simulink model "Wander_Panacea43_1"  (R2019b)
settings: Solver=VariableStepAuto  StartTime=0.0  StopTime=0.5  RelTol=1e-3
values from neighbouring files (symbols this model uses):
  Q = diag([1e-5 1e-5 3])    [panacea_odet.m]    (also in panacea_odet_b.m = diag([1e-2 1e-2 6]); test_kf_simple.m = 0.5)
  R = 0.5*eye(3)    [panacea_odet.m]    (also in panacea_odet_b.m = 0.005*eye(3); test_kf_simple.m = 0.2)
  z = zeros(length(ofdx)*2+3*tracking_delay_length,1,length(out.ofd.time))    [panacea_1.m]    (also in panacea_2.m = zeros(length(ofdx)*2+3*tracking_delay_length+6,1); panacea_3.m = zeros(length(ofdx)*2+3*tracking_delay_length+6,1); panacea_4.m = zeros(length(ofdx)*2+3*tracking_delay_length+6,1); panacea_5.m = zeros(length(ofdx)*2+3*tracking_delay_length+6,1))
undefined symbols (not defined in the file or in its folder): Aa, Add, Ba, Bdd, Cdd, DiscIntNeverNeededParam, f, imuTs, lms, numOfLm, phi, psi, the, x, y
libraries: simulink x9, sharedtransform x2, dspswit3 x1
settings Model: Creator=thinhhoang  LastModifiedBy=thinhhoang
settings OptimizationCC: DefaultParameterBehavior=Inlined  EnhancedBackFolding=on  PassReuseOutputArgsAs=Individual arguments  ZeroExternalMemoryAtStartup=off  ZeroInternalMemoryAtStartup=off  OptimizeBlockOrder=speed  DifferentSizesBufferReuse=on  OptimizationCustomize=off  EfficientTunableParamExpr=on
settings DebuggingCC: ParameterTunabilityLossMsg=error
settings SFSimCC: MATLABDynamicMemAlloc=off
settings RTWCC: SystemTargetFile=ert.tlc  TemplateMakefile=ert_default_tmf  GenerateReport=on  IncludeHyperlinkInReport=on  LaunchReport=on  GenerateTraceInfo=on  GenerateTraceReport=on  GenerateTraceReportSl=on  GenerateTraceReportSf=on  GenerateTraceReportEml=on
settings CodeAppCC: ForceParamTrailComments=on  IgnoreCustomStorageClasses=off  OperatorAnnotations=on  SimulinkDataObjDesc=on  SFDataObjDesc=on  InsertBlockDesc=on
settings ERTTargetCC: TargetLangStandard=C99 (ISO)  GenerateSampleERTMain=on  InlinedParameterPlacement=NonHierarchical  ERTCustomFileTemplate=example_file_process.tlc

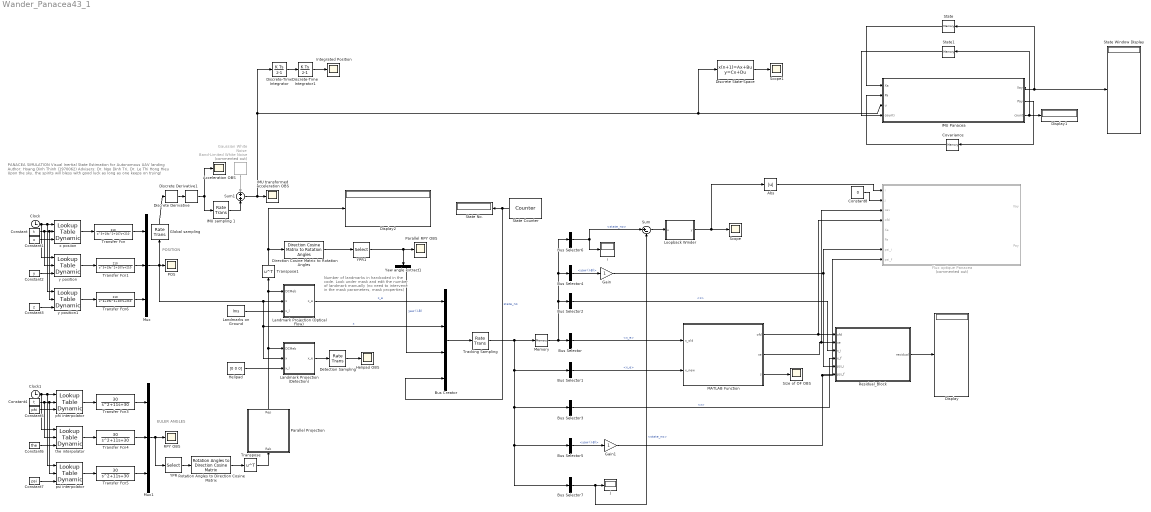
== system Wander_Panacea43_1 ==
  note: PANACEA SIMULATION
      | Visual Inertial State Estimation for Autonomous UAV landing
      | Author: Hoang Dinh Thinh (1970062)
      | Advisers: Dr. Ngo Dinh Tri, Dr. Le Thi Hong Hieu
      | Upon the sky, the spirits will bless with good luck as long as
      | one keeps on trying!
  note: Number of landmarks in hardcoded in the code. Look under mask and edit the number of landmark manually (no need to intervene in the mask parameters, mask properties)
  note: POSITION
  note: EULER ANGLES
  Abs : Abs
  Acceleration OBS : Scope
  Bus Creator : BusCreator  Inputs=4
  Bus Selector : BusSelector  OutputSignals=x_e
  Bus Selector1 : BusSelector  OutputSignals=x_e
  Bus Selector2 : BusSelector  OutputSignals=x
  Bus Selector3 : BusSelector  OutputSignals=x
  Bus Selector4 : BusSelector  OutputSignals=yaw (I-B)
  Bus Selector5 : BusSelector  OutputSignals=yaw (I-B)
  Bus Selector6 : BusSelector  OutputSignals=state_no
  Bus Selector7 : BusSelector  OutputSignals=state_no
  Clock : Clock
  Clock1 : Clock
  Constant : Constant  Value=t
  Constant1 : Constant  Value=x
  Constant2 : Constant  Value=y
  Constant3 : Constant  Value=z
  Constant4 : Constant  Value=t
  Constant5 : Constant  Value=phi
  Constant6 : Constant  Value=the
  Constant7 : Constant  Value=psi
  Constant8 : Constant  Value=0
  Covariance : Memory  InitialCondition=zeros(6,6)
  "Detection Sampling " : RateTransition  OutPortSampleTime=detectionTs
  Direction Cosine Matrix to Rotation Angles : sharedtransform/Direction Cosine Matrix to Rotation Angles  rotationOrder=ZYX  aMode=aMode  action=None  tolerance=eps(2)
      settings: SourceProductName=Aerospace Blockset  SourceProductBaseCode=AE
  Discrete Derivative : simulink/Quick Insert/Discrete/Discrete Derivative  gainval=1.0  ICPrevScaledInput=0.0  OutMin=[]  OutMax=[]  OutDataType=fixdt(1, 16)  OutScaling=2^-10  DoSatur=off
      settings: SourceProductName=Simulink  SourceProductBaseCode=SL
  Discrete Derivative1 : simulink/Quick Insert/Discrete/Discrete Derivative  gainval=1.0  ICPrevScaledInput=0.0  OutMin=[]  OutMax=[]  OutDataType=fixdt(1, 16)  OutScaling=2^-10  DoSatur=off
      settings: SourceProductName=Simulink  SourceProductBaseCode=SL
  Discrete State-Space : DiscreteStateSpace  A=Add  B=Bdd  C=Cdd  D=zeros(3)  SampleTime=-1
  Discrete-Time Integrator : DiscreteIntegrator  SampleTime=-1  ICPrevOutput=DiscIntNeverNeededParam  ICPrevScaledInput=DiscIntNeverNeededParam
  Discrete-Time Integrator1 : DiscreteIntegrator  SampleTime=-1  ICPrevOutput=DiscIntNeverNeededParam  ICPrevScaledInput=DiscIntNeverNeededParam
  Display : Display
  Display1 : Display
  Display2 : Display
  Flux optique Panacea : MATLAB Function  Commented=on  TreatAsAtomicUnit=on  mask{Q=Q, R=R, f=f, Aa=Aa, Ba=Ba}
  Gain : Gain
  Gain1 : Gain
  Gaussian White Noise : simulink/Sources/Band-Limited White Noise  Commented=on  Cov=[1e-3]  Ts=imuTs  seed=[23341]
  Global sampling : RateTransition  OutPortSampleTime=globalTs
  Helipad : Constant  Value=[0 0 0]
  Helipad OBS : Scope
  IMU Panacea : MATLAB Function  TreatAsAtomicUnit=on  SystemSampleTime=imuTs  mask{Q=Q, Aa=Add, Ba=Bdd}
  IMU sampling 1 : RateTransition  OutPortSampleTime=imuTs
  IMU transformed acceleration OBS : Scope
  Integrated Position : Scope
  Landmark Projection (Detection) : MATLAB Function  TreatAsAtomicUnit=on  mask{f=f, numOfLm=1}
      mask prompts: f "Focal length"; numOfLm "Number of landmarks"
  Landmark Projection (Optical Flow) : MATLAB Function  TreatAsAtomicUnit=on  mask{f=f, numOfLm=numOfLm}
      mask prompts: f "Focal length"; numOfLm "Number of landmarks"
  Landmarks on Ground : Constant  Value=lms
  Loopback Winder : MATLAB Function  TreatAsAtomicUnit=on
  MATLAB Function : MATLAB Function  TreatAsAtomicUnit=on
  Memory : Memory  InheritSampleTime=on
  Mux : Mux  Inputs=3
  Mux1 : Mux  Inputs=3
  POS : Scope
  Parallel Projection : MATLAB Function  TreatAsAtomicUnit=on
  Parallel RPY OBS : Scope
  RPY OBS : Scope
  Residual_Block : MATLAB Function  TreatAsAtomicUnit=on  mask{f=f, numOfLm=numOfLm}
      mask prompts: f "Focal length"; numOfLm "Num of LM"
  Rotation Angles to Direction Cosine Matrix : sharedtransform/Rotation Angles to Direction Cosine Matrix  rotationOrder=ZYX  aMode=aMode
      settings: SourceProductBaseCode=AE
  Scope : Scope
  Scope1 : Scope
  Size of OF OBS : Scope
  State : Memory  InitialCondition=zeros(6,1)
  State Counter : dspswit3/Counter  Direction=Up  CountEvent=Free running  CounterSize=User defined  MaxCount=3  InitialCount=0  Output=Count  HitValue=32  ResetInput=on  SamplesPerFrame=1  Ts=imuTs  CntDtype=double  HitDtype=Logical
  State No. : Display
  State Window Display : Display
  State1 : Memory
  Sum : Sum  Inputs=|+-
  Sum1 : Sum  Inputs=+|+
  Tracking Sampling : RateTransition  OutPortSampleTime=trackingTs
  Transfer Fcn : TransferFcn  Numerator=[210]  Denominator=[1 19 107 210]
  Transfer Fcn1 : TransferFcn  Numerator=[210]  Denominator=[1 19 107 210]
  Transfer Fcn3 : TransferFcn  Numerator=[30]  Denominator=[1 11 30]
  Transfer Fcn4 : TransferFcn  Numerator=[30]  Denominator=[1 11 30]
  Transfer Fcn5 : TransferFcn  Numerator=[30]  Denominator=[1 11 30]
  Transfer Fcn6 : TransferFcn  Numerator=[210]  Denominator=[1 19 107 210]
  Transpose : Math  Operator=transpose  SignedPower=off  SaturateOnIntegerOverflow=on
  Transpose1 : Math  Operator=transpose  SignedPower=off  SaturateOnIntegerOverflow=on
  YPR : Selector  InputPortWidth=3  IndexOptions=Index vector (dialog)  Indices=[3 2 1]  OutputSizes=1
  YPR1 : Selector  InputPortWidth=3  IndexOptions=Index vector (dialog)  Indices=[3 2 1]  OutputSizes=1
  Yaw angle extract1 : Demux  Outputs=3
  i : Display
  j : Display
  phi interpolator : simulink/Lookup Tables/Lookup Table Dynamic  LookUpMeth=Interpolation-Use End Values  OutDataType=fixdt('double')  OutScaling=[]  OutputDataTypeScalingMode=Specify via dialog  OutDataTypeStr=double  DoSatur=off
      settings: SourceProductName=Simulink
  psi interpolator : simulink/Lookup Tables/Lookup Table Dynamic  LookUpMeth=Interpolation-Use End Values  OutDataType=fixdt('double')  OutScaling=[]  OutputDataTypeScalingMode=Specify via dialog  OutDataTypeStr=double  DoSatur=off
      settings: SourceProductName=Simulink
  the interpolator : simulink/Lookup Tables/Lookup Table Dynamic  LookUpMeth=Interpolation-Use End Values  OutDataType=fixdt('double')  OutScaling=[]  OutputDataTypeScalingMode=Specify via dialog  OutDataTypeStr=double  DoSatur=off
      settings: SourceProductName=Simulink
  x posiion : simulink/Lookup Tables/Lookup Table Dynamic  LookUpMeth=Interpolation-Use End Values  OutDataType=fixdt('double')  OutScaling=[]  OutputDataTypeScalingMode=Specify via dialog  OutDataTypeStr=double  DoSatur=off
      settings: SourceProductName=Simulink
  y position : simulink/Lookup Tables/Lookup Table Dynamic  LookUpMeth=Interpolation-Use End Values  OutDataType=fixdt('double')  OutScaling=[]  OutputDataTypeScalingMode=Specify via dialog  OutDataTypeStr=double  DoSatur=off
      settings: SourceProductName=Simulink
  y position1 : simulink/Lookup Tables/Lookup Table Dynamic  LookUpMeth=Interpolation-Use End Values  OutDataType=fixdt('double')  OutScaling=[]  OutputDataTypeScalingMode=Specify via dialog  OutDataTypeStr=double  DoSatur=off
      settings: SourceProductName=Simulink
  wires:
  Clock/1 -> y position/1, y position1/1, x posiion/1
  Constant/1 -> y position/2, y position1/2, x posiion/2
  Constant1/1 -> x posiion/3
  Constant2/1 -> y position/3
  Constant3/1 -> y position1/3
  x posiion/1 -> Transfer Fcn/1
  Transfer Fcn/1 -> Mux/1
  Mux/1 -> Global sampling/1, Landmark Projection (Detection)/2(x), Bus Creator/2, Landmark Projection (Optical Flow)/2(x), POS/1  "x"
  Clock1/1 -> the interpolator/1, psi interpolator/1, phi interpolator/1
  Constant4/1 -> the interpolator/2, psi interpolator/2, phi interpolator/2
  Constant5/1 -> phi interpolator/3
  Constant6/1 -> the interpolator/3
  Constant7/1 -> psi interpolator/3
  phi interpolator/1 -> Transfer Fcn3/1
  the interpolator/1 -> Transfer Fcn4/1
  psi interpolator/1 -> Transfer Fcn5/1
  Transfer Fcn3/1 -> Mux1/1
  Transfer Fcn4/1 -> Mux1/2
  Transfer Fcn5/1 -> Mux1/3
  Mux1/1 -> YPR/1, RPY OBS/1
  YPR/1 -> Rotation Angles to Direction Cosine Matrix/1
  Rotation Angles to Direction Cosine Matrix/1 -> Transpose/1
  Landmarks on Ground/1 -> Landmark Projection (Optical Flow)/3(x_l)
  Transpose/1 -> Parallel Projection/1(Reb)
  Parallel Projection/1(Rep) -> Landmark Projection (Detection)/1(DCMeb), Landmark Projection (Optical Flow)/1(DCMeb), Transpose1/1
  Transpose1/1 -> Display2/1, Direction Cosine Matrix to Rotation Angles/1
  Direction Cosine Matrix to Rotation Angles/1 -> YPR1/1
  YPR1/1 -> Yaw angle extract1/1, Parallel RPY OBS/1
  Discrete Derivative/1 -> Discrete Derivative1/1
  Discrete Derivative1/1 -> IMU sampling 1/1, Acceleration OBS/1
  Transfer Fcn1/1 -> Mux/2
  y position/1 -> Transfer Fcn1/1
  y position1/1 -> Transfer Fcn6/1
  Transfer Fcn6/1 -> Mux/3
  Gaussian White Noise/1 -> Sum1/1
  MATLAB Function/3(s) -> Size of OF OBS/1
  Helipad/1 -> Landmark Projection (Detection)/3(x_l)
  Landmark Projection (Detection)/1(x_e) -> "Detection Sampling "/1
  "Detection Sampling "/1 -> Helipad OBS/1
  IMU sampling 1/1 -> Sum1/2
  Global sampling/1 -> Discrete Derivative/1
  Landmark Projection (Optical Flow)/1(x_e) -> Bus Creator/1  "x_e"
  Bus Creator/1 -> Tracking Sampling/1
  Tracking Sampling/1 -> Bus Selector7/1, Bus Selector5/1, Bus Selector3/1, Bus Selector1/1, Memory/1
  Memory/1 -> Bus Selector6/1, Bus Selector4/1, Bus Selector2/1, Bus Selector/1
  Bus Selector/1 -> MATLAB Function/1(x_old)  "<x_e>"
  Bus Selector1/1 -> MATLAB Function/2(x_new)  "<x_e>"
  MATLAB Function/1(ofd) -> Flux optique Panacea/4(ofd), Residual_Block/1(ofd)
  MATLAB Function/2(xe) -> Flux optique Panacea/3(xev), Residual_Block/2(xe)
  Bus Selector2/1 -> Residual_Block/3(x_i)  "<x>"
  Bus Selector3/1 -> Residual_Block/4(x_f)  "<x>"
  Bus Selector4/1 -> Gain/1  "<yaw (I-B)>"
  Bus Selector5/1 -> Gain1/1  "<yaw (I-B)>"
  Residual_Block/1(residual) -> Display/1
  Gain/1 -> Residual_Block/5(psi_i), Flux optique Panacea/7(psi_i)
  Gain1/1 -> Flux optique Panacea/8(psi_f), Residual_Block/6(psi_f)
  Yaw angle extract1/3 -> Bus Creator/3  "yaw (I-B)"
  State Counter/1 -> Bus Creator/4, State No./1  "state_no"
  Bus Selector6/1 -> Sum/1, i/1  "<state_no>"
  Bus Selector7/1 -> Sum/2, j/1  "<state_no>"
  Sum/1 -> Loopback Winder/1(u)
  Loopback Winder/1(y) -> Abs/1, Scope/1
  Constant8/1 -> Flux optique Panacea/2(j)
  Abs/1 -> Flux optique Panacea/1(i)
  State/1 -> IMU Panacea/1(Xa)
  Covariance/1 -> IMU Panacea/2(Pa)
  Sum1/1 -> Discrete State-Space/1, IMU Panacea/3(u), Discrete-Time Integrator/1, IMU transformed acceleration OBS/1
  IMU Panacea/1(Xay) -> State/1, State Window Display/1
  IMU Panacea/2(Pay) -> Covariance/1
  Discrete-Time Integrator/1 -> Discrete-Time Integrator1/1
  Discrete-Time Integrator1/1 -> Integrated Position/1
  Discrete State-Space/1 -> Scope1/1
  IMU Panacea/3(count) -> Display1/1, State1/1
  State1/1 -> IMU Panacea/4(counti)

== matlab function Wander_Panacea43_1/Parallel Projection ==
  data: Reb input; Rep output
function Rep = ParallelProjection(Reb)
Rpb = ParallelProject(Reb);
Rep = Rpb'*Reb;
end

== matlab function Wander_Panacea43_1/Landmark Projection (Optical Flow) ==
  data: DCMeb input size=[3 3]; x input size=[1 3]; x_l input size=[numOfLm 3]; x_e output size=[numOfLm 2]; f parameter size=1
function x_e  = pi(DCMeb, x, x_l, f)
    numOfLm = length(x_l);
    x_e = zeros(numOfLm, 2);
    for i=1:numOfLm
        x_e(i,:) = Project(f, DCMeb, x, x_l(i,:));
    end
end

== matlab function Wander_Panacea43_1/MATLAB Function ==
  data: x_old input; ofd output; xe output; x_new input; s output size=1
function [ofd, xe, s] = OpticalFlowEstimator(x_old, x_new)
    numOfLm = length(x_old);
    ofd = zeros(numOfLm, 2);
    k = 0;
    for i=1:numOfLm
        if (x_old(i,1)==-1 || x_old(i,2)==-1 || x_new(i,1)==-1 || x_new(i,2)==-1)
            ofd(i,:) = [0 0];
        else
            ofd(i,:) = x_new(i,:) - x_old(i,:);
            k = k+1;
        end
    end
    s = k;
    xe = x_old;
end

== matlab function Wander_Panacea43_1/Residual_Block ==
  data: ofd input; xe input; residual output; x_i input; x_f input; psi_i input; psi_f input; f parameter
function residual = fcn(ofd,xe,x_i,x_f,psi_i,psi_f,f)
    numOfLm = length(ofd);
    % All psi angle: I-B
    result = -ones(1,length(ofd)*2);
    for i = 1:numOfLm
        if (ofd(i,1)==0 || ofd(i,2)==0)
            % skip
        else
            r = Measurement(f,xe(i,1),xe(i,2),ofd(i,1),ofd(i,2),-psi_i,-psi_f,x_i,x_f);
            result(i*2-1) = r(1);
            result(i*2) = r(2);
        end
    end
    residual = result;
end

== matlab function Wander_Panacea43_1/Landmark Projection (Detection) ==
  data: DCMeb input size=[3 3]; x input size=[1 3]; x_l input size=[numOfLm 3]; x_e output size=[numOfLm 2]; f parameter size=1; numOfLm parameter size=1
function x_e  = pi(DCMeb, x, x_l, f, numOfLm)
    x_e = zeros(1, 2);
    for i=1:numOfLm
        x_e(i,:) = Project(f, DCMeb, x, x_l(i,:));
    end
end

== matlab function Wander_Panacea43_1/Loopback Winder ==
  data: u input; y output
function y = Loopback(u)
if u>0
    y=-3;
else
    y=u;
end

== matlab function Wander_Panacea43_1/Flux optique Panacea ==
  data: i input; Xay output; j input; xev input; ofd input; Xa input; Pa input; psi_i input; psi_f input; R parameter; f parameter; Pay output; Aa parameter
function [Xay,Pay] = PanaceaOFSM(i,j,xev,ofd,Xa,Pa,psi_i,psi_f,R,f,Aa)
N_window = length(Xa)/6 - 2;
[Xay, Pay] = PanaceaOF(i,j,xev,ofd,psi_i,psi_f,Xa,Pa,R,f,N_window,Aa);
end

== matlab function Wander_Panacea43_1/IMU Panacea ==
  data: Xa input; Pa input; u input; Xay output; Pay output; Q parameter; Aa parameter; Ba parameter; counti input; count output
function [Xay,Pay,count] = PanaceaAccel(Xa,Pa,u, Q, Aa, Ba,counti)
[Xay,Pay] = PanaceaIMU(Xa,Pa,Q,Aa,Ba,u);
count = counti + 1;
end
